simulink model "sim_1"  (R2021b)
settings: Solver=VariableStepAuto  StartTime=0.0  StopTime=2.8  RelTol=1e-3
values from neighbouring files (symbols this model uses):
  lambda0 = tc.lambda0_tc    [gnrt_tc.m]
  r0 = tc.r0_tc    [gnrt_tc.m]
  v_lam0 = tc.v_lam0_tc    [gnrt_tc.m]
  v_r0 = tc.v_r0_tc    [gnrt_tc.m]
  zeta = tc.zeta_tc    [gnrt_tc.m]
settings Model: SimulationMode=rapid-accelerator  Creator=kusha  LastModifiedBy=kusha

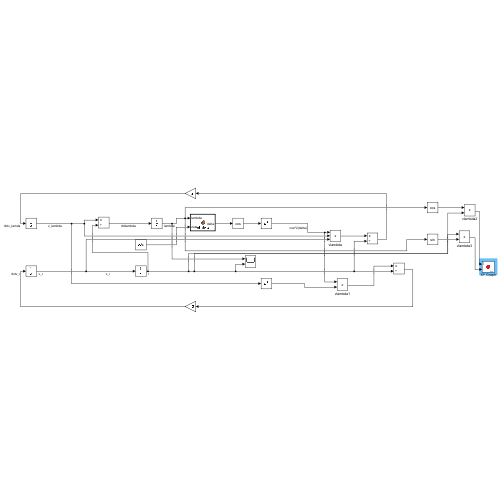
[thumbnail: Simulink's stored preview of the top-level diagram]
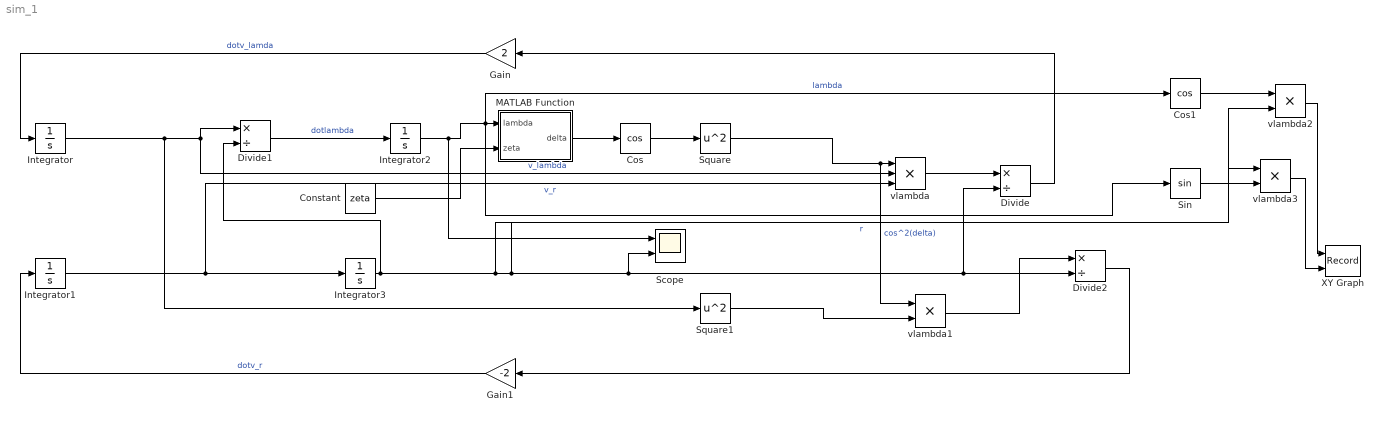
== system sim_1 ==
  Constant : Constant  Value=zeta
  Cos : Trigonometry  Operator=cos
  Cos1 : Trigonometry  Operator=cos
  Divide : Product  Inputs=*/
  Divide1 : Product  Inputs=*/
  Divide2 : Product  Inputs=*/
  Gain : Gain  Gain=2
  Gain1 : Gain  Gain=-2
  Integrator : Integrator  InitialCondition=v_lam0
  Integrator1 : Integrator  InitialCondition=v_r0
  Integrator2 : Integrator  InitialCondition=lambda0
  Integrator3 : Integrator  InitialCondition=r0
  MATLAB Function : MATLAB Function  TreatAsAtomicUnit=on
  Scope : Scope  NumInputPorts=2
  Sin : Trigonometry
  Square : Math  Operator=square  SaturateOnIntegerOverflow=on
  Square1 : Math  Operator=square  SaturateOnIntegerOverflow=on
  XY Graph : Record  FileSettingsInternal="{\"entries\":[{\"content\":{\"excelSettings\":{\"content\":{},\"type\":\"Streamout.ExcelSettings\"}},\"type\":\"Streamout.FileSettingStorage\",\"uuid\":\"eb0dca59-41fc-47a4-a85b-fb932ed385e0\"}],\"packageUris\":[\"http://schema.mathworks.com/mf0/streamout_blocks/R2020a\"],\"version\":\"1.0\"}"  Layout=[1 1]  SignalsInternal="{\"entries\":[{\"content\":{\"signals\":[{\"content\":{\"blockPath\":[\"sim/XY Graph\"],\"channel\":[],\"dimensions\":[1],\"domain\":\"sim/XY Graph\",\"lineColor\":\"#a2142f\",\"plots\":[1],\"port\":1,\"sid\":[\"\"],\"signalID\":354,\"signalName\":\"vlambda2\"},\"type\":\"RecordBlkView.Signal\",\"uuid\":\"2eec6901-5751-4e48-88b2-d0f87884e2de\"},{\"content\":{\"blockPath\":[\"sim/XY Graph\"],\"channel\":[],\"dimensions\":[1],\"domain\":\"sim/XY Graph\",\"lineColor\":\"#139fff\",\"plots\":[1],\"port\":2,\"sid\":[\"\"],\"signalID\":358,\"signalName\":\"vlambda3\"},\"type\":\"RecordBlkView.Signal\",\"uuid\":\"79773e6a-4977-44cd-b7ad-c6f217099482\"}]},\"type\":\"RecordBlkView.InputSignals\",\"uuid\":\"10a08504-caf4-483c-8ff5-3754a1d4b3e8\"}],\"packageUris\":[\"http://schema.mathworks.com/mf0/streamout_blocks/R2020a\"],\"version\":\"1.0\"}"  VisualizationBindings="{\"xyplotplugin\":{\"info\":[{\"series\":[{\"bindingParametersList\":[{\"parameter\":\"X-Axis\",\"signalID\":354,\"signalName\":\"vlambda2\"},{\"parameter\":\"Y-Axis\",\"signalID\":358,\"signalName\":\"vlambda3\"}],\"seriesID\":13232}],\"subplotID\":1}]}}"  CompatibilityTag=XY
  vlambda : Product  Inputs=3
  vlambda1 : Product
  vlambda2 : Product
  vlambda3 : Product
  wires:
  Integrator/1 -> Square1/1, Divide1/1, vlambda/2  "v_lambda"
  Gain/1 -> Integrator/1  "dotv_lamda"
  Gain1/1 -> Integrator1/1  "dotv_r"
  Integrator1/1 -> Integrator3/1, vlambda/3  "v_r"
  Divide1/1 -> Integrator2/1  "dotlambda"
  Integrator2/1 -> Scope/1, Cos1/1, MATLAB Function/1(lambda), Sin/1  "lambda"
  Integrator3/1 -> Divide1/2, vlambda2/2, vlambda3/1, Scope/2, Divide2/2, Divide/2  "r"
  MATLAB Function/1(delta) -> Cos/1
  Cos/1 -> Square/1
  Square/1 -> vlambda1/1, vlambda/1  "cos^2(delta)"
  vlambda/1 -> Divide/1
  Divide/1 -> Gain/1
  Square1/1 -> vlambda1/2
  vlambda1/1 -> Divide2/1
  Divide2/1 -> Gain1/1
  Constant/1 -> MATLAB Function/2(zeta)
  Cos1/1 -> vlambda2/1
  Sin/1 -> vlambda3/2
  vlambda2/1 -> XY Graph/1
  vlambda3/1 -> XY Graph/2

== matlab function sim_1/MATLAB Function ==
  data: lambda input; delta output; zeta input
function delta = ret_delta(lambda, zeta)
delta = atan(2*(lambda - zeta));
